simulink library "headingSetpointCaclulation"  (R2018a)
settings: Solver=VariableStepAuto  StartTime=0.0  StopTime=10.0  RelTol=1e-3
settings Model: Creator=mitch  LastModifiedBy=mitch

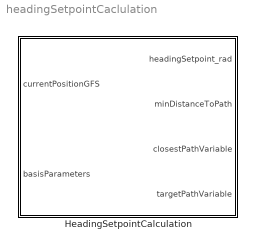
== system headingSetpointCaclulation ==
  HeadingSetpointCalculation : Subsystem  mask{searchDistance=0, tol=0, meanElev=0, leadLength=0, initialPathVariable=0}
      mask prompts: searchDistance "Search Distance"; tol "Tolerance"; meanElev "Mean Elevation [Deg]"; leadLength "Lead Length"; initialPathVariable "Initial Path Variable"

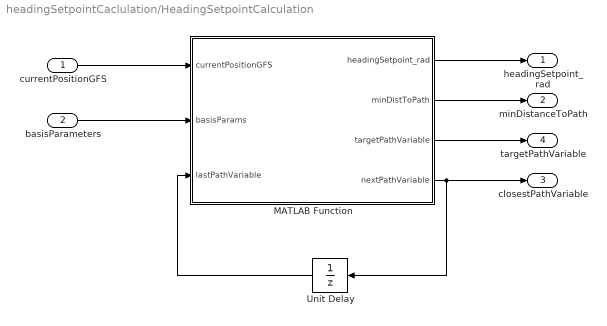
== system headingSetpointCaclulation/HeadingSetpointCalculation ==
  currentPositionGFS : Inport
  basisParameters : Inport  Port=2
  MATLAB Function : MATLAB Function  TreatAsAtomicUnit=on
  Unit Delay : UnitDelay  InitialCondition=initialPathVariable  SampleTime=-1
  headingSetpoint_rad : Outport
  minDistanceToPath : Outport  Port=2
  closestPathVariable : Outport  Port=3
  targetPathVariable : Outport  Port=4
  wires:
  currentPositionGFS/1 -> MATLAB Function/1(currentPositionGFS)
  basisParameters/1 -> MATLAB Function/2(basisParams)
  Unit Delay/1 -> MATLAB Function/3(lastPathVariable)
  MATLAB Function/4(nextPathVariable) -> Unit Delay/1, closestPathVariable/1
  MATLAB Function/1(headingSetpoint_rad) -> headingSetpoint_rad/1
  MATLAB Function/2(minDistToPath) -> minDistanceToPath/1
  MATLAB Function/3(targetPathVariable) -> targetPathVariable/1

== matlab function headingSetpointCaclulation/HeadingSetpointCalculation/MATLAB Function ==
  data: currentPositionGFS input; headingSetpoint_rad output; minDistToPath output; targetPathVariable output; basisParams input; lastPathVariable input; nextPathVariable output; searchDistance parameter; tol parameter; meanElev parameter; leadLength parameter
function [headingSetpoint_rad,minDistToPath,targetPathVariable,nextPathVariable] = ...
    getHeadingSetpoint(currentPositionGFS,...
    basisParams,lastPathVariable, searchDistance, tol, meanElev, leadLength)

meanElev = meanElev*pi/180;

[nextPathVariable,minDistToPath] = ...
    pathProjection(currentPositionGFS,basisParams,meanElev,...
    lastPathVariable,searchDistance,tol);

nextPathVariable = rem(nextPathVariable,1);

targetPathVariable = nextPathVariable+leadLength;
%  targetPathVariable = nextPathVariable;

[azStar,znStar] = pathShape(basisParams,meanElev,targetPathVariable);

lat1 = pi/2-currentPositionGFS(3);
lon1 = currentPositionGFS(2);

lat2 = pi/2 - znStar;
lon2 = azStar;

sp = pi/2-greatcircleaz(lat1, lon1, lat2, lon2);
headingSetpoint_rad = mod(sp+pi,2*pi)-pi; % wrap to [-pi pi]

end

function az = greatcircleaz(lat1,lon1,lat2,lon2)

% Inputs LAT1, LON1, LAT2, LON2 are in units of radians.
% First equation on this page:
% https://en.wikipedia.org/wiki/Great-circle_navigation
az = atan2(cos(lat2) .* sin(lon2-lon1),...
    cos(lat1) .* sin(lat2) - sin(lat1) .* cos(lat2) .* cos(lon2-lon1));

end


function d = distanceToPath(currentPositionGFS,bp,meanElev,s)
% https://en.wikipedia.org/wiki/Great-circle_distance
% Uses first vectorized version from this website
[azimuth,zenith] = pathShape(bp,meanElev,s);
r1s = [currentPositionGFS(1) azimuth zenith];
r2s = [currentPositionGFS(1) currentPositionGFS(2) currentPositionGFS(3)];

r1c = [r1s(1)*cos(r1s(2))*sin(r1s(3)) ...
    r1s(1)*sin(r1s(2))*sin(r1s(3)) ...
    r1s(1)*cos(r1s(3))];

r2c = [r2s(1)*cos(r2s(2))*sin(r2s(3)) ...
    r2s(1)*sin(r2s(2))*sin(r2s(3)) ...
    r2s(1)*cos(r2s(3))];

n1 = r1c./norm(r1c);
n2 = r2c./norm(r2c);

deltaSigma = acos(dot(n1,n2));
d = currentPositionGFS(1)*deltaSigma;


%
% lambda1 = azimuth;
% phi1    = pi/2-zenith;
%
% lambda2 = currentPositionGFS(2);
% phi2    = pi/2-currentPositionGFS(3);
%
%
% dp = phi2-phi1;
% dl = lambda2-lambda1;
%
% deltaSigma = 2*asin(sqrt(sin(dp/2)^2+cos(phi1)*cos(phi2)*sin(dl/2)^2));
%
% d = currentPositionGFS(1)*deltaSigma;

end

function [xStar,fMin] = pathProjection(currentPositionGFS,bp,meanElev,...
    lastPathVariable,searchDistance,tol)

gr = (sqrt(5) - 1) / 2;

x = [0 0 0 0];
x(1) = lastPathVariable;
x(4) = lastPathVariable+searchDistance;
x(3) = x(1) + (x(4)-x(1))*gr;
x(2) = x(4) - (x(4)-x(1))*gr;

f = [0 0 0 0];
f(1) =  distanceToPath(currentPositionGFS,bp,meanElev,x(1));
f(2) =  distanceToPath(currentPositionGFS,bp,meanElev,x(2));
f(3) =  distanceToPath(currentPositionGFS,bp,meanElev,x(3));
f(4) =  distanceToPath(currentPositionGFS,bp,meanElev,x(4));
for ii = 1:1000
    if x(4) - x(1) < tol
        break
    end
    if f(2)<f(3)
        x = [x(1) ...
            x(3)-(x(3)-x(1))*gr...
            x(2:3)];
        f = [f(1) ...
            distanceToPath(currentPositionGFS,bp,meanElev,x(2))...
            f(2:3)];
        
    else %f(3)<f(2)
        x = [x(2:3) ...
            x(2)+(x(4)-x(2))*gr...
            x(4)];
        f = [f(2:3) ...
            distanceToPath(currentPositionGFS,bp,meanElev,x(3))...
            f(4)];
    end
    
end

[xStar,idx] = min(x);
fMin  = f(idx);

end
